simulink model "Atmosphere_Model"  (R2023b)
settings: Solver=VariableStepAuto  StartTime=0.0  StopTime=10.0  RelTol=1e-3
settings Model: Creator=atzml  LastModifiedBy=atzml

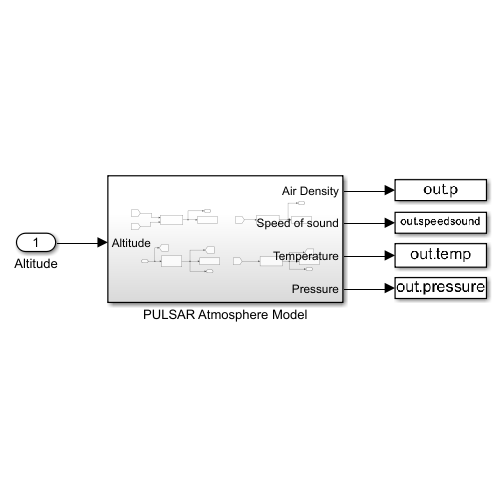
[thumbnail: Simulink's stored preview of the top-level diagram]
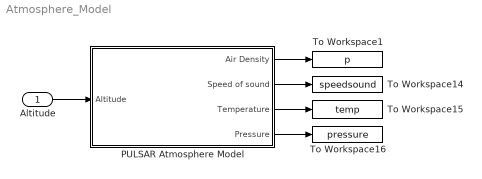
== system Atmosphere_Model ==
  Altitude : Inport
  PULSAR Atmosphere Model : Subsystem
  To Workspace1 : ToWorkspace  VariableName=p  SaveFormat=Timeseries  SampleTime=-1
  To Workspace14 : ToWorkspace  VariableName=speedsound  SaveFormat=Timeseries  SampleTime=-1
  To Workspace15 : ToWorkspace  VariableName=temp  SaveFormat=Timeseries  SampleTime=-1
  To Workspace16 : ToWorkspace  VariableName=pressure  SaveFormat=Timeseries  SampleTime=-1
  wires:
  PULSAR Atmosphere Model/4(Pressure) -> To Workspace16/1
  PULSAR Atmosphere Model/2(Speed of sound) -> To Workspace14/1
  Altitude/1 -> PULSAR Atmosphere Model/1(Altitude)
  PULSAR Atmosphere Model/1(Air Density) -> To Workspace1/1
  PULSAR Atmosphere Model/3(Temperature) -> To Workspace15/1

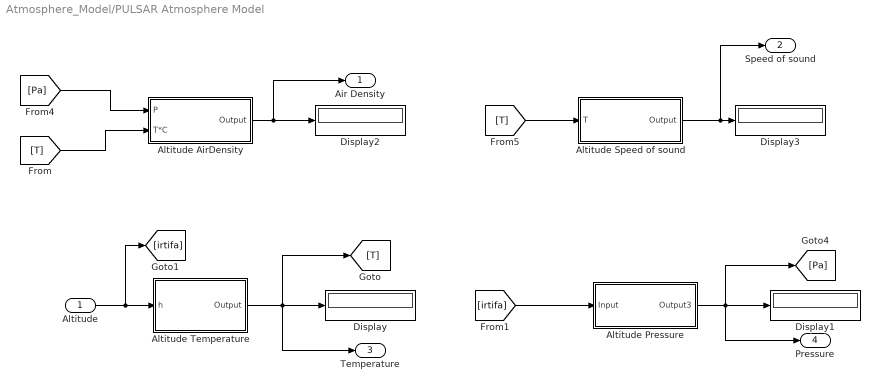
== system Atmosphere_Model/PULSAR Atmosphere Model ==
  Altitude : Inport
  Altitude AirDensity : Subsystem
  Altitude Pressure : Subsystem
  Altitude Speed of sound : Subsystem
  Altitude Temperature : Subsystem
  Display{,1..3} (4 alike) : Display
  Air Density : Outport
  Speed of sound : Outport  Port=2
  Temperature : Outport  Port=3
  Pressure : Outport  Port=4
  wires:
  [irtifa] -> Altitude Pressure/1(Input)
  Altitude AirDensity/1(Output) -> Air Density/1, Display2/1
  Altitude/1 -> [irtifa], Altitude Temperature/1(h)
  Altitude Speed of sound/1(Output) -> Speed of sound/1, Display3/1
  Altitude Temperature/1(Output) -> Temperature/1, Display/1, [T]
  [Pa] -> Altitude AirDensity/1(P)
  Altitude Pressure/1(Output3) -> Pressure/1, Display1/1, [Pa]
  [T] -> Altitude Speed of sound/1(T)
  [T] -> Altitude AirDensity/2(T*C)

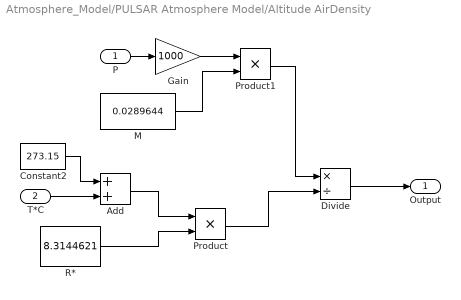
== system Atmosphere_Model/PULSAR Atmosphere Model/Altitude AirDensity ==
  P : Inport
  T*C : Inport  Port=2
  Add : Sum
  Constant2 : Constant  Value=273.15
  Divide : Product  Inputs=*/
  Gain : Gain  Gain=1000
  M : Constant  Value=0.0289644
  Product : Product
  Product1 : Product
  R* : Constant  Value=8.3144621
  Output : Outport
  wires:
  M/1 -> Product1/2
  R*/1 -> Product/2
  Divide/1 -> Output/1
  P/1 -> Gain/1
  Constant2/1 -> Add/1
  Product/1 -> Divide/2
  Product1/1 -> Divide/1
  Gain/1 -> Product1/1
  T*C/1 -> Add/2
  Add/1 -> Product/1

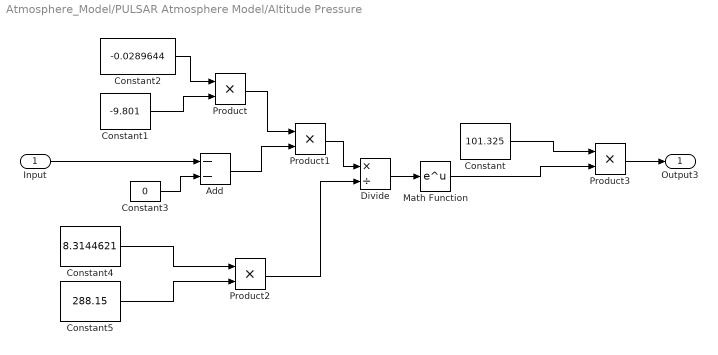
== system Atmosphere_Model/PULSAR Atmosphere Model/Altitude Pressure ==
  Input : Inport
  Add : Sum  Inputs=--
  Constant : Constant  Value=101.325
  Constant1 : Constant  Value=-9.801
  Constant2 : Constant  Value=-0.0289644
  Constant3 : Constant  Value=0
  Constant4 : Constant  Value=8.3144621
  Constant5 : Constant  Value=288.15
  Divide : Product  Inputs=*/
  Math Function : Math
  Product{,1..3} (4 alike) : Product
  Output3 : Outport
  wires:
  Constant2/1 -> Product/1
  Constant1/1 -> Product/2
  Input/1 -> Add/1
  Constant3/1 -> Add/2
  Add/1 -> Product1/2
  Product/1 -> Product1/1
  Constant4/1 -> Product2/1
  Constant5/1 -> Product2/2
  Product1/1 -> Divide/1
  Product2/1 -> Divide/2
  Divide/1 -> Math Function/1
  Constant/1 -> Product3/1
  Math Function/1 -> Product3/2
  Product3/1 -> Output3/1

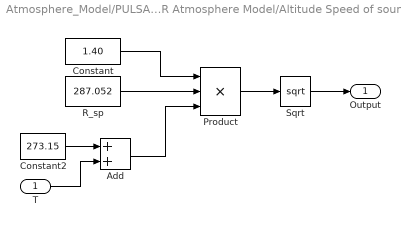
== system Atmosphere_Model/PULSAR Atmosphere Model/Altitude Speed of sound ==
  T : Inport
  Add : Sum
  Constant : Constant  Value=1.40
  Constant2 : Constant  Value=273.15
  Product : Product  Inputs=3
  R_sp : Constant  Value=287.052
  Sqrt : Sqrt
  Output : Outport
  wires:
  Constant2/1 -> Add/1
  T/1 -> Add/2
  Constant/1 -> Product/1
  R_sp/1 -> Product/2
  Add/1 -> Product/3
  Product/1 -> Sqrt/1
  Sqrt/1 -> Output/1

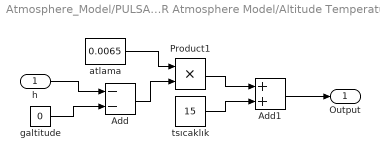
== system Atmosphere_Model/PULSAR Atmosphere Model/Altitude Temperature ==
  h : Inport
  Add : Sum  Inputs=--
  Add1 : Sum
  Product1 : Product
  atlama : Constant  Value=0.0065
  galtitude : Constant  Value=0
  tsıcaklık : Constant  Value=15
  Output : Outport
  wires:
  Product1/1 -> Add1/1
  galtitude/1 -> Add/2
  Add1/1 -> Output/1
  Add/1 -> Product1/2
  tsıcaklık/1 -> Add1/2
  h/1 -> Add/1
  atlama/1 -> Product1/1
